simulink model "ForwardDyn_CTC_SCARA_Trajectory"  (R2023a)
settings: Solver=FixedStepAuto  StartTime=0.0  StopTime=10  FixedStep=0.01  RelTol=1e-3
libraries: slpidlib x4
settings Model: Creator=abdom  LastModifiedBy=abdom

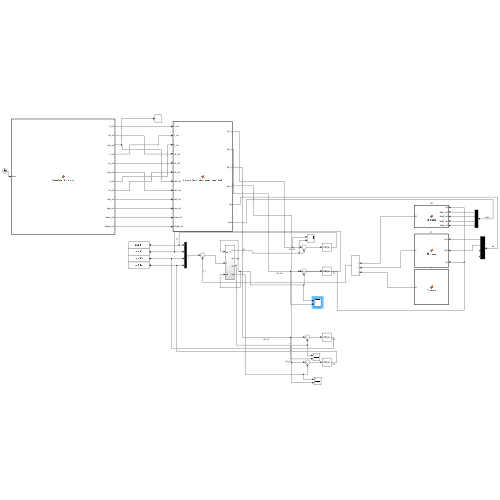
[thumbnail: Simulink's stored preview of the top-level diagram]
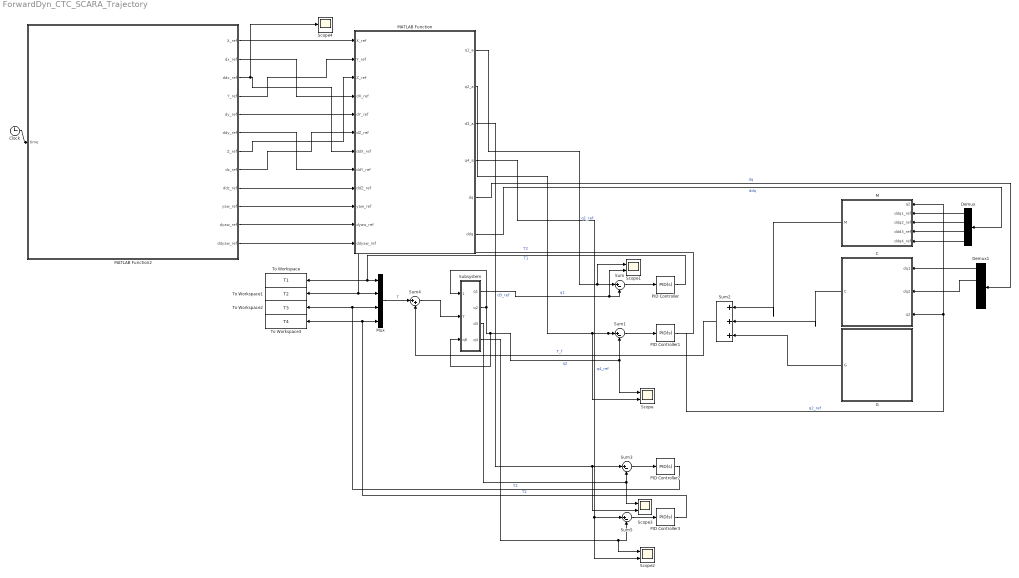
== system ForwardDyn_CTC_SCARA_Trajectory ==
  C : MATLAB Function  TreatAsAtomicUnit=on
  Clock : Clock
  Demux : Demux
  Demux1 : Demux
  G : MATLAB Function  TreatAsAtomicUnit=on
  M : MATLAB Function  TreatAsAtomicUnit=on
  MATLAB Function : MATLAB Function  TreatAsAtomicUnit=on
  MATLAB Function2 : MATLAB Function  TreatAsAtomicUnit=on
  Mux : Mux
  PID Controller : slpidlib/PID Controller  Controller=PID  Form=Parallel  TimeDomain=Continuous-time  UseExternalTs=off  SampleTime=-1  IntegratorMethod=Forward Euler  FilterMethod=Forward Euler  ControllerParametersSource=internal  P=50  I=10  UseKiTs=off  D=10  N=100  UseFilter=on  TunerSelectOption=Transfer Function Based (PID Tuner App)  InitialConditionSource=internal  InitialConditionForIntegrator=0  InitialConditionForFilter=0  DifferentiatorICPrevScaledInput=0  ExternalReset=none  TrackingMode=off  Kt=1  LimitOutput=off  SatLimitsSource=internal  UpperSaturationLimit=inf  LowerSaturationLimit=-inf  LinearizeAsGain=on  AntiWindupMode=none  Kb=1  LimitIntegrator=off  UpperIntegratorSaturationLimit=inf  LowerIntegratorSaturationLimit=-inf  POutMin=[]  POutMax=[]  IOutMin=[]  IOutMax=[]  DOutMin=[]  DOutMax=[]  NOutMin=[]  NOutMax=[]  SumOutMin=[]  SumOutMax=[]  SaturationOutMin=[]  SaturationOutMax=[]  PParamMin=[]  PParamMax=[]  IParamMin=[]  IParamMax=[]  DParamMin=[]  DParamMax=[]  NParamMin=[]  NParamMax=[]  KbParamMin=[]  KbParamMax=[]  KtParamMin=[]  KtParamMax=[]  KbOutMin=[]  KbOutMax=[]  KtOutMin=[]  KtOutMax=[]  IntegratorOutMin=[]  IntegratorOutMax=[]  FilterOutMin=[]  FilterOutMax=[]  SumI1OutMin=[]  SumI1OutMax=[]  SumI2OutMin=[]  SumI2OutMax=[]  SumI3OutMin=[]  SumI3OutMax=[]  SumI4OutMin=[]  SumI4OutMax=[]  SumDOutMin=[]  SumDOutMax=[]  DifferentiatorOutMin=[]  DifferentiatorOutMax=[]  FilterDiffOutCoefMin=[]  FilterDiffOutCoefMax=[]  ReciprocalOutMin=[]  ReciprocalOutMax=[]  SumDenOutMin=[]  SumDenOutMax=[]  SumNumOutMin=[]  SumNumOutMax=[]  DivideOutMin=[]  DivideOutMax=[]  UdiffTsProdOutMin=[]  UdiffTsProdOutMax=[]  NTsProdOutMin=[]  NTsProdOutMax=[]  UintegralTsProdOutMin=[]  UintegralTsProdOutMax=[]  UngainTsProdOutMin=[]  UngainTsProdOutMax=[]  ClampingZeroOutDataTypeStr=Inherit: Inherit via back propagation  ClampingZeroOutMin=[]  ClampingZeroOutMax=[]  FilterDenConstantOutDataTypeStr=Inherit: Inherit via back propagation  FilterDenConstantOutMin=[]  FilterDenConstantOutMax=[]  PCopyOutDataTypeStr=Inherit: Inherit via back propagation  PCopyOutMin=[]  PCopyOutMax=[]  NCopyOutDataTypeStr=Inherit: Inherit via back propagation  NCopyOutMin=[]  NCopyOutMax=[]  IntegratorContinuousStateAttributes=''  IntegratorStateMustResolveToSignalObject=off  IntegratorRTWStateStorageClass=Auto  FilterContinuousStateAttributes=''  FilterStateMustResolveToSignalObject=off  FilterRTWStateStorageClass=Auto  ParallelPVariant=InternalParameters  IdealPVariant=Disabled  IVariant=InternalParameters  DVariant=InternalParameters  IntegratorVariant=Continuous  SatVariant=Disabled  AWVariant=Passthrough  PCopyVariant=Disabled  TRVariant=Disabled  FdbkBlocksVariant=Forward  IdealPFdbkVariant=Disabled  SatFdbkVariant=Disabled  DerivativeFilterVariant=ContFilter  NVariant=InternalParameters  NCopyVariant=Disabled  FilterICVariant=InternalICsFilter  IntegratorICVariant=InternalICs  ExternalResetVariant=Disabled  TRSumVariant=Passthrough  SumFdbkVariant=Disabled  SumVariant=Sum_PID  TsampFilterVariant=InternalTs  TsampNgainVariant=Passthrough  TsampIntegralVariant=Disabled_SignalSpec  ExternalSaturationOutDataTypeStr=Inherit: Same as second input
  PID Controller1 : slpidlib/PID Controller  Controller=PID  Form=Parallel  TimeDomain=Continuous-time  UseExternalTs=off  SampleTime=-1  IntegratorMethod=Forward Euler  FilterMethod=Forward Euler  ControllerParametersSource=internal  P=500  I=100  UseKiTs=off  D=50  N=1  UseFilter=on  TunerSelectOption=Transfer Function Based (PID Tuner App)  InitialConditionSource=internal  InitialConditionForIntegrator=0  InitialConditionForFilter=0  DifferentiatorICPrevScaledInput=0  ExternalReset=none  TrackingMode=off  Kt=1  LimitOutput=off  SatLimitsSource=internal  UpperSaturationLimit=inf  LowerSaturationLimit=-inf  LinearizeAsGain=on  AntiWindupMode=none  Kb=1  LimitIntegrator=off  UpperIntegratorSaturationLimit=inf  LowerIntegratorSaturationLimit=-inf  POutMin=[]  POutMax=[]  IOutMin=[]  IOutMax=[]  DOutMin=[]  DOutMax=[]  NOutMin=[]  NOutMax=[]  SumOutMin=[]  SumOutMax=[]  SaturationOutMin=[]  SaturationOutMax=[]  PParamMin=[]  PParamMax=[]  IParamMin=[]  IParamMax=[]  DParamMin=[]  DParamMax=[]  NParamMin=[]  NParamMax=[]  KbParamMin=[]  KbParamMax=[]  KtParamMin=[]  KtParamMax=[]  KbOutMin=[]  KbOutMax=[]  KtOutMin=[]  KtOutMax=[]  IntegratorOutMin=[]  IntegratorOutMax=[]  FilterOutMin=[]  FilterOutMax=[]  SumI1OutMin=[]  SumI1OutMax=[]  SumI2OutMin=[]  SumI2OutMax=[]  SumI3OutMin=[]  SumI3OutMax=[]  SumI4OutMin=[]  SumI4OutMax=[]  SumDOutMin=[]  SumDOutMax=[]  DifferentiatorOutMin=[]  DifferentiatorOutMax=[]  FilterDiffOutCoefMin=[]  FilterDiffOutCoefMax=[]  ReciprocalOutMin=[]  ReciprocalOutMax=[]  SumDenOutMin=[]  SumDenOutMax=[]  SumNumOutMin=[]  SumNumOutMax=[]  DivideOutMin=[]  DivideOutMax=[]  UdiffTsProdOutMin=[]  UdiffTsProdOutMax=[]  NTsProdOutMin=[]  NTsProdOutMax=[]  UintegralTsProdOutMin=[]  UintegralTsProdOutMax=[]  UngainTsProdOutMin=[]  UngainTsProdOutMax=[]  ClampingZeroOutDataTypeStr=Inherit: Inherit via back propagation  ClampingZeroOutMin=[]  ClampingZeroOutMax=[]  FilterDenConstantOutDataTypeStr=Inherit: Inherit via back propagation  FilterDenConstantOutMin=[]  FilterDenConstantOutMax=[]  PCopyOutDataTypeStr=Inherit: Inherit via back propagation  PCopyOutMin=[]  PCopyOutMax=[]  NCopyOutDataTypeStr=Inherit: Inherit via back propagation  NCopyOutMin=[]  NCopyOutMax=[]  IntegratorContinuousStateAttributes=''  IntegratorStateMustResolveToSignalObject=off  IntegratorRTWStateStorageClass=Auto  FilterContinuousStateAttributes=''  FilterStateMustResolveToSignalObject=off  FilterRTWStateStorageClass=Auto  ParallelPVariant=InternalParameters  IdealPVariant=Disabled  IVariant=InternalParameters  DVariant=InternalParameters  IntegratorVariant=Continuous  SatVariant=Disabled  AWVariant=Passthrough  PCopyVariant=Disabled  TRVariant=Disabled  FdbkBlocksVariant=Forward  IdealPFdbkVariant=Disabled  SatFdbkVariant=Disabled  DerivativeFilterVariant=ContFilter  NVariant=InternalParameters  NCopyVariant=Disabled  FilterICVariant=InternalICsFilter  IntegratorICVariant=InternalICs  ExternalResetVariant=Disabled  TRSumVariant=Passthrough  SumFdbkVariant=Disabled  SumVariant=Sum_PID  TsampFilterVariant=InternalTs  TsampNgainVariant=Passthrough  TsampIntegralVariant=Disabled_SignalSpec  ExternalSaturationOutDataTypeStr=Inherit: Same as second input
  PID Controller2 : slpidlib/PID Controller  Controller=PID  Form=Parallel  TimeDomain=Continuous-time  UseExternalTs=off  SampleTime=-1  IntegratorMethod=Forward Euler  FilterMethod=Forward Euler  ControllerParametersSource=internal  P=500  I=100  UseKiTs=off  D=5  N=1  UseFilter=on  TunerSelectOption=Transfer Function Based (PID Tuner App)  InitialConditionSource=internal  InitialConditionForIntegrator=0  InitialConditionForFilter=0  DifferentiatorICPrevScaledInput=0  ExternalReset=none  TrackingMode=off  Kt=1  LimitOutput=off  SatLimitsSource=internal  UpperSaturationLimit=inf  LowerSaturationLimit=-inf  LinearizeAsGain=on  AntiWindupMode=none  Kb=1  LimitIntegrator=off  UpperIntegratorSaturationLimit=inf  LowerIntegratorSaturationLimit=-inf  POutMin=[]  POutMax=[]  IOutMin=[]  IOutMax=[]  DOutMin=[]  DOutMax=[]  NOutMin=[]  NOutMax=[]  SumOutMin=[]  SumOutMax=[]  SaturationOutMin=[]  SaturationOutMax=[]  PParamMin=[]  PParamMax=[]  IParamMin=[]  IParamMax=[]  DParamMin=[]  DParamMax=[]  NParamMin=[]  NParamMax=[]  KbParamMin=[]  KbParamMax=[]  KtParamMin=[]  KtParamMax=[]  KbOutMin=[]  KbOutMax=[]  KtOutMin=[]  KtOutMax=[]  IntegratorOutMin=[]  IntegratorOutMax=[]  FilterOutMin=[]  FilterOutMax=[]  SumI1OutMin=[]  SumI1OutMax=[]  SumI2OutMin=[]  SumI2OutMax=[]  SumI3OutMin=[]  SumI3OutMax=[]  SumI4OutMin=[]  SumI4OutMax=[]  SumDOutMin=[]  SumDOutMax=[]  DifferentiatorOutMin=[]  DifferentiatorOutMax=[]  FilterDiffOutCoefMin=[]  FilterDiffOutCoefMax=[]  ReciprocalOutMin=[]  ReciprocalOutMax=[]  SumDenOutMin=[]  SumDenOutMax=[]  SumNumOutMin=[]  SumNumOutMax=[]  DivideOutMin=[]  DivideOutMax=[]  UdiffTsProdOutMin=[]  UdiffTsProdOutMax=[]  NTsProdOutMin=[]  NTsProdOutMax=[]  UintegralTsProdOutMin=[]  UintegralTsProdOutMax=[]  UngainTsProdOutMin=[]  UngainTsProdOutMax=[]  ClampingZeroOutDataTypeStr=Inherit: Inherit via back propagation  ClampingZeroOutMin=[]  ClampingZeroOutMax=[]  FilterDenConstantOutDataTypeStr=Inherit: Inherit via back propagation  FilterDenConstantOutMin=[]  FilterDenConstantOutMax=[]  PCopyOutDataTypeStr=Inherit: Inherit via back propagation  PCopyOutMin=[]  PCopyOutMax=[]  NCopyOutDataTypeStr=Inherit: Inherit via back propagation  NCopyOutMin=[]  NCopyOutMax=[]  IntegratorContinuousStateAttributes=''  IntegratorStateMustResolveToSignalObject=off  IntegratorRTWStateStorageClass=Auto  FilterContinuousStateAttributes=''  FilterStateMustResolveToSignalObject=off  FilterRTWStateStorageClass=Auto  ParallelPVariant=InternalParameters  IdealPVariant=Disabled  IVariant=InternalParameters  DVariant=InternalParameters  IntegratorVariant=Continuous  SatVariant=Disabled  AWVariant=Passthrough  PCopyVariant=Disabled  TRVariant=Disabled  FdbkBlocksVariant=Forward  IdealPFdbkVariant=Disabled  SatFdbkVariant=Disabled  DerivativeFilterVariant=ContFilter  NVariant=InternalParameters  NCopyVariant=Disabled  FilterICVariant=InternalICsFilter  IntegratorICVariant=InternalICs  ExternalResetVariant=Disabled  TRSumVariant=Passthrough  SumFdbkVariant=Disabled  SumVariant=Sum_PID  TsampFilterVariant=InternalTs  TsampNgainVariant=Passthrough  TsampIntegralVariant=Disabled_SignalSpec  ExternalSaturationOutDataTypeStr=Inherit: Same as second input
  PID Controller3 : slpidlib/PID Controller  Controller=PID  Form=Parallel  TimeDomain=Continuous-time  UseExternalTs=off  SampleTime=-1  IntegratorMethod=Forward Euler  FilterMethod=Forward Euler  ControllerParametersSource=internal  P=500  I=200  UseKiTs=off  D=10  N=1  UseFilter=on  TunerSelectOption=Transfer Function Based (PID Tuner App)  InitialConditionSource=internal  InitialConditionForIntegrator=0  InitialConditionForFilter=0  DifferentiatorICPrevScaledInput=0  ExternalReset=none  TrackingMode=off  Kt=1  LimitOutput=off  SatLimitsSource=internal  UpperSaturationLimit=inf  LowerSaturationLimit=-inf  LinearizeAsGain=on  AntiWindupMode=none  Kb=1  LimitIntegrator=off  UpperIntegratorSaturationLimit=inf  LowerIntegratorSaturationLimit=-inf  POutMin=[]  POutMax=[]  IOutMin=[]  IOutMax=[]  DOutMin=[]  DOutMax=[]  NOutMin=[]  NOutMax=[]  SumOutMin=[]  SumOutMax=[]  SaturationOutMin=[]  SaturationOutMax=[]  PParamMin=[]  PParamMax=[]  IParamMin=[]  IParamMax=[]  DParamMin=[]  DParamMax=[]  NParamMin=[]  NParamMax=[]  KbParamMin=[]  KbParamMax=[]  KtParamMin=[]  KtParamMax=[]  KbOutMin=[]  KbOutMax=[]  KtOutMin=[]  KtOutMax=[]  IntegratorOutMin=[]  IntegratorOutMax=[]  FilterOutMin=[]  FilterOutMax=[]  SumI1OutMin=[]  SumI1OutMax=[]  SumI2OutMin=[]  SumI2OutMax=[]  SumI3OutMin=[]  SumI3OutMax=[]  SumI4OutMin=[]  SumI4OutMax=[]  SumDOutMin=[]  SumDOutMax=[]  DifferentiatorOutMin=[]  DifferentiatorOutMax=[]  FilterDiffOutCoefMin=[]  FilterDiffOutCoefMax=[]  ReciprocalOutMin=[]  ReciprocalOutMax=[]  SumDenOutMin=[]  SumDenOutMax=[]  SumNumOutMin=[]  SumNumOutMax=[]  DivideOutMin=[]  DivideOutMax=[]  UdiffTsProdOutMin=[]  UdiffTsProdOutMax=[]  NTsProdOutMin=[]  NTsProdOutMax=[]  UintegralTsProdOutMin=[]  UintegralTsProdOutMax=[]  UngainTsProdOutMin=[]  UngainTsProdOutMax=[]  ClampingZeroOutDataTypeStr=Inherit: Inherit via back propagation  ClampingZeroOutMin=[]  ClampingZeroOutMax=[]  FilterDenConstantOutDataTypeStr=Inherit: Inherit via back propagation  FilterDenConstantOutMin=[]  FilterDenConstantOutMax=[]  PCopyOutDataTypeStr=Inherit: Inherit via back propagation  PCopyOutMin=[]  PCopyOutMax=[]  NCopyOutDataTypeStr=Inherit: Inherit via back propagation  NCopyOutMin=[]  NCopyOutMax=[]  IntegratorContinuousStateAttributes=''  IntegratorStateMustResolveToSignalObject=off  IntegratorRTWStateStorageClass=Auto  FilterContinuousStateAttributes=''  FilterStateMustResolveToSignalObject=off  FilterRTWStateStorageClass=Auto  ParallelPVariant=InternalParameters  IdealPVariant=Disabled  IVariant=InternalParameters  DVariant=InternalParameters  IntegratorVariant=Continuous  SatVariant=Disabled  AWVariant=Passthrough  PCopyVariant=Disabled  TRVariant=Disabled  FdbkBlocksVariant=Forward  IdealPFdbkVariant=Disabled  SatFdbkVariant=Disabled  DerivativeFilterVariant=ContFilter  NVariant=InternalParameters  NCopyVariant=Disabled  FilterICVariant=InternalICsFilter  IntegratorICVariant=InternalICs  ExternalResetVariant=Disabled  TRSumVariant=Passthrough  SumFdbkVariant=Disabled  SumVariant=Sum_PID  TsampFilterVariant=InternalTs  TsampNgainVariant=Passthrough  TsampIntegralVariant=Disabled_SignalSpec  ExternalSaturationOutDataTypeStr=Inherit: Same as second input
  Scope{,1..3} (4 alike) : Scope  NumInputPorts=2
  Scope4 : Scope
  Subsystem : Subsystem
  Sum{,1,3,5} (4 alike) : Sum  Inputs=|+-
  Sum2 : Sum  Inputs=|+++
  Sum4 : Sum  Inputs=|++
  To Workspace : ToWorkspace  VariableName=T1  SampleTime=-1
  To Workspace1 : ToWorkspace  VariableName=T2  SampleTime=-1
  To Workspace2 : ToWorkspace  VariableName=T3  SampleTime=-1
  To Workspace3 : ToWorkspace  VariableName=T4  SampleTime=-1
  wires:
  PID Controller/1 -> To Workspace/1, Mux/1  "T1"
  Subsystem/1(q1) -> Scope1/2, Sum/2  "q1"
  Subsystem/2(q2) -> Subsystem/3(q8), Scope/1, Sum1/2, Subsystem/1(q2_2)  "q2"
  MATLAB Function/1(q1_a) -> Scope1/1, Sum/1  "q1_ref"
  MATLAB Function/2(q2_a) -> C/3(q2), M/1(q2), Sum1/1, Scope/2  "q2_ref"
  Sum/1 -> PID Controller/1
  Sum1/1 -> PID Controller1/1
  PID Controller1/1 -> Mux/2, To Workspace1/1  "T2"
  Mux/1 -> Sum4/1  "T"
  Sum2/1 -> Sum4/2  "T_f"
  Sum4/1 -> Subsystem/2(T)
  M/1(M) -> Sum2/1
  G/1(G) -> Sum2/3
  C/1(C) -> Sum2/2
  Subsystem/3(d3) -> Scope3/1, Sum3/2
  Subsystem/4(q4) -> Scope2/1, Sum5/2
  MATLAB Function/4(q4_a) -> Scope2/2, Sum5/1  "q4_ref"
  MATLAB Function/3(d3_a) -> Scope3/2, Sum3/1  "d3_ref"
  Sum3/1 -> PID Controller2/1
  Sum5/1 -> PID Controller3/1
  PID Controller2/1 -> Mux/3, To Workspace2/1  "T2"
  PID Controller3/1 -> Mux/4, To Workspace3/1  "T2"
  Clock/1 -> MATLAB Function2/1(time)
  MATLAB Function/5(dq) -> Demux1/1  "dq"
  MATLAB Function/6(ddq) -> Demux/1  "ddq"
  Demux/1 -> M/2(ddq1_ref)
  Demux/2 -> M/3(ddq2_ref)
  Demux/4 -> M/5(ddq4_ref)
  Demux/3 -> M/4(ddd3_ref)
  Demux1/1 -> C/1(dq1)
  Demux1/2 -> C/2(dq2)
  MATLAB Function2/4(Y_ref) -> MATLAB Function/2(Y_ref)
  MATLAB Function2/2(dx_ref) -> MATLAB Function/4(dX_ref)
  MATLAB Function2/3(ddx_ref) -> Scope4/1, MATLAB Function/7(ddX_ref)
  MATLAB Function2/5(dy_ref) -> MATLAB Function/5(dY_ref)
  MATLAB Function2/6(ddy_ref) -> MATLAB Function/8(ddY_ref)
  MATLAB Function2/7(Z_ref) -> MATLAB Function/3(Z_ref)
  MATLAB Function2/8(dz_ref) -> MATLAB Function/6(dZ_ref)
  MATLAB Function2/9(ddz_ref) -> MATLAB Function/9(ddZ_ref)
  MATLAB Function2/10(yaw_ref) -> MATLAB Function/10(yaw_ref)
  MATLAB Function2/11(dyaw_ref) -> MATLAB Function/11(dyaw_ref)
  MATLAB Function2/12(ddyaw_ref) -> MATLAB Function/12(ddyaw_ref)
  MATLAB Function2/1(X_ref) -> MATLAB Function/1(X_ref)

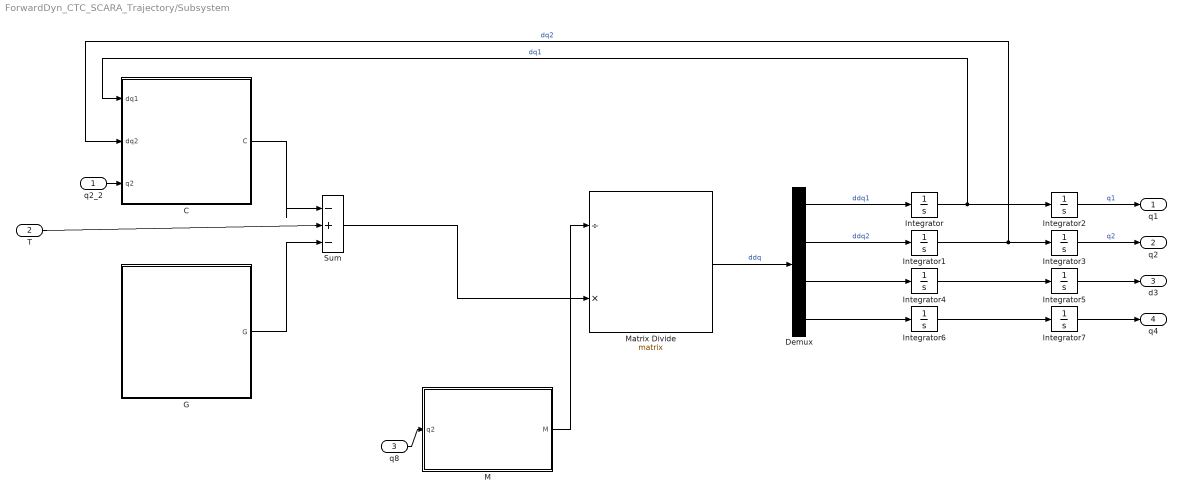
== system ForwardDyn_CTC_SCARA_Trajectory/Subsystem ==
  q2_2 : Inport
  T : Inport  Port=2
  q8 : Inport  Port=3
  C : MATLAB Function  TreatAsAtomicUnit=on
  Demux : Demux
  G : MATLAB Function  TreatAsAtomicUnit=on
  Integrator{,1..7} (8 alike) : Integrator
  M : MATLAB Function  TreatAsAtomicUnit=on
  Matrix Divide : Product  Inputs=/*  Multiplication=Matrix(*)
  Sum : Sum  Inputs=|-+-
  q1 : Outport
  q2 : Outport  Port=2
  d3 : Outport  Port=3
  q4 : Outport  Port=4
  wires:
  G/1(G) -> Sum/3
  Matrix Divide/1 -> Demux/1  "ddq"
  Integrator1/1 -> C/2(dq2), Integrator3/1  "dq2"
  Integrator/1 -> C/1(dq1), Integrator2/1  "dq1"
  Sum/1 -> Matrix Divide/2
  C/1(C) -> Sum/1
  T/1 -> Sum/2
  Demux/1 -> Integrator/1  "ddq1"
  Demux/2 -> Integrator1/1  "ddq2"
  q8/1 -> M/1(q2)
  M/1(M) -> Matrix Divide/1
  Integrator2/1 -> q1/1  "q1"
  q2_2/1 -> C/3(q2)
  Integrator3/1 -> q2/1  "q2"
  Demux/3 -> Integrator4/1
  Integrator4/1 -> Integrator5/1
  Integrator5/1 -> d3/1
  Integrator7/1 -> q4/1
  Integrator6/1 -> Integrator7/1
  Demux/4 -> Integrator6/1

== matlab function ForwardDyn_CTC_SCARA_Trajectory/MATLAB Function2 ==
  data: X_ref output; dx_ref output; ddx_ref output; time input; Y_ref output; dy_ref output; ddy_ref output; Z_ref output; dz_ref output; ddz_ref output; yaw_ref output; dyaw_ref output; ddyaw_ref output
function [X_ref, dx_ref, ddx_ref, Y_ref, dy_ref, ddy_ref, Z_ref, dz_ref, ddz_ref, yaw_ref, dyaw_ref, ddyaw_ref] = Trajectory_Generator(time)
    % Trajectory settings
    Tspan = 10;
    % Position
    x0 = 0.6; xf = 0.9;
    y0 = 0; yf = 0;
    z0 = 0; zf = 0.1;
    yaw0 = 0.1; yawf = 0.2;
    
    % Velocity (start/end at rest)
    dx0 = 0; dxf = 0;
    dy0 = 0; dyf = 0;
    dz0 = 0; dzf = 0;
    dyaw0 = 0; dyawf = 0;
    
    % Acceleration (no initial jerk)
    ddx0 = 0; ddxf = 0;
    ddy0 = 0; ddyf = 0;
    ddz0 = 0; ddzf = 0;
    ddyaw0 = 0; ddyawf = 0;

    % Compute only inside trajectory span
    if time < 0 || time > Tspan
        X_ref = 0;
        dx_ref = 0;
        ddx_ref = 0;
        Y_ref = 0;
        dy_ref = 0;
        ddy_ref = 0;
        Z_ref = 0;
        dz_ref = 0;
        ddz_ref = 0;
        yaw_ref = 0;
        dyaw_ref = 0;
        ddyaw_ref = 0;
    else
        % Precomputed coefficients
        n0 = x0;
        n1 = dx0;
        n2 = ddx0 / 2;
        n3 = ddxf/(2*Tspan) - (3*ddx0)/(2*Tspan) - (6*dx0)/Tspan^2 - (4*dxf)/Tspan^2 - (10*x0)/Tspan^3 + (10*xf)/Tspan^3;
        n4 = (3*ddx0)/(2*Tspan^2) - ddxf/Tspan^2 + (8*dx0)/Tspan^3 + (7*dxf)/Tspan^3 + (15*x0)/Tspan^4 - (15*xf)/Tspan^4;
        n5 = ddxf/(2*Tspan^3) - ddx0/(2*Tspan^3) - (3*dx0)/Tspan^4 - (3*dxf)/Tspan^4 - (6*x0)/Tspan^5 + (6*xf)/Tspan^5;

        % Compute position, velocity, acceleration
        X_ref = n0 + n1*time + n2*time^2 + n3*time^3 + n4*time^4 + n5*time^5;
        dx_ref = n1 + 2*n2*time + 3*n3*time^2 + 4*n4*time^3 + 5*n5*time^4;
        ddx_ref = 2*n2 + 6*n3*time + 12*n4*time^2 + 20*n5*time^3;

        n0 = y0;
        n1 = dy0;
        n2 = ddy0 / 2;
        n3 = ddyf/(2*Tspan) - (3*ddy0)/(2*Tspan) - (6*dy0)/Tspan^2 - (4*dyf)/Tspan^2 - (10*y0)/Tspan^3 + (10*yf)/Tspan^3;
        n4 = (3*ddy0)/(2*Tspan^2) - ddyf/Tspan^2 + (8*dy0)/Tspan^3 + (7*dyf)/Tspan^3 + (15*y0)/Tspan^4 - (15*yf)/Tspan^4;
        n5 = ddyf/(2*Tspan^3) - ddy0/(2*Tspan^3) - (3*dy0)/Tspan^4 - (3*dyf)/Tspan^4 - (6*y0)/Tspan^5 + (6*yf)/Tspan^5;
        Y_ref = n0 + n1*time + n2*time^2 + n3*time^3 + n4*time^4 + n5*time^5;
        dy_ref = n1 + 2*n2*time + 3*n3*time^2 + 4*n4*time^3 + 5*n5*time^4;
        ddy_ref = 2*n2 + 6*n3*time + 12*n4*time^2 + 20*n5*time^3;

        n0 = z0;
        n1 = dz0;
        n2 = ddz0 / 2;
        n3 = ddzf/(2*Tspan) - (3*ddz0)/(2*Tspan) - (6*dz0)/Tspan^2 - (4*dzf)/Tspan^2 - (10*z0)/Tspan^3 + (10*zf)/Tspan^3;
        n4 = (3*ddz0)/(2*Tspan^2) - ddzf/Tspan^2 + (8*dz0)/Tspan^3 + (7*dzf)/Tspan^3 + (15*z0)/Tspan^4 - (15*zf)/Tspan^4;
        n5 = ddzf/(2*Tspan^3) - ddz0/(2*Tspan^3) - (3*dz0)/Tspan^4 - (3*dzf)/Tspan^4 - (6*z0)/Tspan^5 + (6*zf)/Tspan^5;
        Z_ref = n0 + n1*time + n2*time^2 + n3*time^3 + n4*time^4 + n5*time^5;
        dz_ref = n1 + 2*n2*time + 3*n3*time^2 + 4*n4*time^3 + 5*n5*time^4;
        ddz_ref = 2*n2 + 6*n3*time + 12*n4*time^2 + 20*n5*time^3;

        n0 = yaw0;
        n1 = dyaw0;
        n2 = ddyaw0 / 2;
        n3 = ddyawf/(2*Tspan) - (3*ddyaw0)/(2*Tspan) - (6*dyaw0)/Tspan^2 - (4*dyawf)/Tspan^2 - (10*yaw0)/Tspan^3 + (10*yawf)/Tspan^3;
        n4 = (3*ddyaw0)/(2*Tspan^2) - ddyawf/Tspan^2 + (8*dyaw0)/Tspan^3 + (7*dyawf)/Tspan^3 + (15*yaw0)/Tspan^4 - (15*yawf)/Tspan^4;
        n5 = ddyawf/(2*Tspan^3) - ddyaw0/(2*Tspan^3) - (3*dyaw0)/Tspan^4 - (3*dyawf)/Tspan^4 - (6*yaw0)/Tspan^5 + (6*yawf)/Tspan^5;

        yaw_ref = n0 + n1*time + n2*time^2 + n3*time^3 + n4*time^4 + n5*time^5;
        dyaw_ref = n1 + 2*n2*time + 3*n3*time^2 + 4*n4*time^3 + 5*n5*time^4;
        ddyaw_ref = 2*n2 + 6*n3*time + 12*n4*time^2 + 20*n5*time^3;


    end
end

== matlab function ForwardDyn_CTC_SCARA_Trajectory/Subsystem/C ==
  data: dq1 input; C output; dq2 input; q2 input
function C = C_scara(dq1,dq2,q2)
%C_scara
%    C = C_scara(L2,L3,DQ1,DQ2,M2,M3,M4,Q2)

%    This function was generated by the Symbolic Math Toolbox version 9.3.
%    12-May-2025 16:21:30
L2 = 0.6;
L3 = 0.4;
m2 = 3.0;
m3 = 2.5;
m4 = 1.0;


t2 = sin(q2);
t3 = m3.*2.0;
t4 = m4.*2.0;
t5 = m2+t3+t4;
C = [L2.*L3.*dq2.*t2.*t5.*(dq1.*2.0+dq2).*(-1.0./2.0);(L2.*L3.*dq1.^2.*t2.*t5)./2.0;0.0;0.0];
end

== matlab function ForwardDyn_CTC_SCARA_Trajectory/Subsystem/M ==
  data: M output; q2 input
function M = M_scara(q2)
%M_scara
%    M = M_scara(Izz1,Izz2,Izz4,L2,L3,M1,M2,M3,M4,Q2)

%    This function was generated by the Symbolic Math Toolbox version 9.3.
%    12-May-2025 16:21:29


L2 = 0.6;
L3 = 0.4;
m1 = 5.0;
m2 = 3.0;
m3 = 2.5;
m4 = 1.0;
Izz1 = 0.20;
Izz2 = 0.08;
Izz4 = 0.02;


t2 = cos(q2);
t3 = L2.^2;
t4 = L3.^2;
t5 = m3.*t4;
t6 = m4.*t4;
t7 = L2.*L3.*m3.*t2;
t8 = L2.*L3.*m4.*t2;
t9 = (m2.*t4)./4.0;
t10 = (L2.*L3.*m2.*t2)./2.0;
t11 = Izz2+Izz4+t5+t6+t7+t8+t9+t10;
M = reshape([Izz1+Izz2+Izz4+t5+t6+t7.*2.0+t8.*2.0+t9+(m1.*t3)./4.0+m2.*t3+m3.*t3+m4.*t3+L2.*L3.*m2.*t2,t11,0.0,Izz4,t11,Izz2+Izz4+t5+t6+t9,0.0,Izz4,0.0,0.0,m3./4.0+m4,0.0,Izz4,Izz4,0.0,Izz4],[4,4]);
end

== matlab function ForwardDyn_CTC_SCARA_Trajectory/Subsystem/G ==
  data: G output
function G = G_scara()
%G_scara
%    G = G_scara(M3,M4)

%    This function was generated by the Symbolic Math Toolbox version 9.3.
%    12-May-2025 16:21:30

m3 = 2.5;
m4 = 1.0;


G = [0.0;0.0;m3.*(9.81e+2./2.0e+2)+m4.*(9.81e+2./1.0e+2);0.0];
end

== matlab function ForwardDyn_CTC_SCARA_Trajectory/G ==
  data: G output
function G = G_scara()
%G_scara
%    G = G_scara(M3,M4)

%    This function was generated by the Symbolic Math Toolbox version 9.3.
%    12-May-2025 16:21:30

m3 = 2.5;
m4 = 1.0;


G = [0.0;0.0;m3.*(9.81e+2./2.0e+2)+m4.*(9.81e+2./1.0e+2);0.0];
end

== matlab function ForwardDyn_CTC_SCARA_Trajectory/C ==
  data: dq1 input; C output; dq2 input; q2 input
function C = C_scara(dq1,dq2,q2)
%C_scara
%    C = C_scara(L2,L3,DQ1,DQ2,M2,M3,M4,Q2)

%    This function was generated by the Symbolic Math Toolbox version 9.3.
%    12-May-2025 16:21:30
L2 = 0.6;
L3 = 0.4;
m2 = 3.0;
m3 = 2.5;
m4 = 1.0;


t2 = sin(q2);
t3 = m3.*2.0;
t4 = m4.*2.0;
t5 = m2+t3+t4;
C = [L2.*L3.*dq2.*t2.*t5.*(dq1.*2.0+dq2).*(-1.0./2.0);(L2.*L3.*dq1.^2.*t2.*t5)./2.0;0.0;0.0];
end

== matlab function ForwardDyn_CTC_SCARA_Trajectory/M ==
  data: M output; q2 input; ddq1_ref input; ddq2_ref input; ddd3_ref input; ddq4_ref input
function M = M_scara(q2, ddq1_ref, ddq2_ref, ddd3_ref, ddq4_ref)
%M_scara
%    M = M_scara(Izz1,Izz2,Izz4,L2,L3,M1,M2,M3,M4,Q2)

%    This function was generated by the Symbolic Math Toolbox version 9.3.
%    12-May-2025 16:21:29


L2 = 0.6;
L3 = 0.4;
m1 = 5.0;
m2 = 3.0;
m3 = 2.5;
m4 = 1.0;
Izz1 = 0.20;
Izz2 = 0.08;
Izz4 = 0.02;


t2 = cos(q2);
t3 = L2.^2;
t4 = L3.^2;
t5 = m3.*t4;
t6 = m4.*t4;
t7 = L2.*L3.*m3.*t2;
t8 = L2.*L3.*m4.*t2;
t9 = (m2.*t4)./4.0;
t10 = (L2.*L3.*m2.*t2)./2.0;
t11 = Izz2+Izz4+t5+t6+t7+t8+t9+t10;
M_final = reshape([Izz1+Izz2+Izz4+t5+t6+t7.*2.0+t8.*2.0+t9+(m1.*t3)./4.0+m2.*t3+m3.*t3+m4.*t3+L2.*L3.*m2.*t2,t11,0.0,Izz4,t11,Izz2+Izz4+t5+t6+t9,0.0,Izz4,0.0,0.0,m3./4.0+m4,0.0,Izz4,Izz4,0.0,Izz4],[4,4]);
M = M_final * [ddq1_ref ddq2_ref ddd3_ref ddq4_ref]'; 
end

== matlab function ForwardDyn_CTC_SCARA_Trajectory/MATLAB Function ==
  data: X_ref input; q1_a output; Y_ref input; Z_ref input; dX_ref input; dY_ref input; dZ_ref input; ddX_ref input; ddY_ref input; ddZ_ref input; q2_a output; d3_a output; q4_a output; yaw_ref input; dyaw_ref input; ddyaw_ref input; dq output; ddq output
function [q1_a, q2_a, d3_a, q4_a, dq, ddq] = inverse_Kinematics_scara_analytical( ...
    X_ref, Y_ref, Z_ref, dX_ref, dY_ref, dZ_ref, ddX_ref, ddY_ref, ddZ_ref, ...
    yaw_ref, dyaw_ref, ddyaw_ref)

    % Link lengths
    L1 = 0.4;
    L2 = 0.6;
    L3 = 0.4;
    L5 = 0.1;

    %% Inverse Position Kinematics (q1, q2, d3)
    x = X_ref;
    y = Y_ref;
    z = Z_ref;

    r2 = x^2 + y^2;
    cos_q2 = (r2 - L2^2 - L3^2) / (2 * L2 * L3);
    sin_q2 = sqrt(1 - cos_q2^2);  % Elbow-down
    q2 = atan2(sin_q2, cos_q2);

    k1 = L2 + L3 * cos_q2;
    k2 = L3 * sin_q2;
    q1 = atan2(y, x) - atan2(k2, k1);

    d3 = z - L1 - L5;

    %% Orientation handling (q4)
    % Maintain desired orientation: q4 = yaw_ref - q1 - q2
    q4 = yaw_ref - q1 - q2;

    %% Jacobian (3x3 for [q1 q2 d3])
    J = [ ...
        -L2*sin(q1) - L3*sin(q1 + q2), -L3*sin(q1 + q2), 0; ...
         L2*cos(q1) + L3*cos(q1 + q2),  L3*cos(q1 + q2), 0; ...
         0,                            0,               1 ...
    ];

    %% Joint velocities
    dp = [dX_ref; dY_ref; dZ_ref];
    dq_temp = pinv(J) * dp;
    dq1 = dq_temp(1); dq2 = dq_temp(2); dd3 = dq_temp(3);

    % q4 velocity
    dq4 = dyaw_ref - dq1 - dq2;

    dq = [dq1; dq2; dd3; dq4];

    %% Jacobian derivative (J_dot)
    J_dot = [ ...
        -L2*cos(q1)*dq1 - L3*cos(q1 + q2)*(dq1 + dq2), -L3*cos(q1 + q2)*(dq1 + dq2), 0; ...
        -L2*sin(q1)*dq1 - L3*sin(q1 + q2)*(dq1 + dq2), -L3*sin(q1 + q2)*(dq1 + dq2), 0; ...
         0, 0, 0 ...
    ];

    %% Joint accelerations
    ddp = [ddX_ref; ddY_ref; ddZ_ref];
    ddq_temp = pinv(J) * (ddp - J_dot * dq_temp);

    ddq1 = ddq_temp(1); ddq2 = ddq_temp(2); ddd3 = ddq_temp(3);
    ddq4 = ddyaw_ref - ddq1 - ddq2;

    ddq = [ddq1; ddq2; ddd3; ddq4];

    %% Output joint positions
    q1_a = q1;
    q2_a = q2;
    d3_a = d3;
    q4_a = q4;
end
